simulink model "Event4_2018a"  (R2018a)
settings: Solver=FixedStepDiscrete  StartTime=0.0  StopTime=0.1  FixedStep=0.1  RelTol=1e-3  EnableMultiTasking=on
settings Model: Creator=BEAR  LastModifiedBy=apple
settings SolverCC: AutoInsertRateTranBlk=on
settings DataIOCC: LimitDataPoints=on
settings OptimizationCC: LifeSpan=inf
settings DebuggingCC: AllowSymbolicDim=off  SFUnexpectedBacktrackingDiag=warning  SFNoUnconditionalDefaultTransitionDiag=warning  SFExecutionAtInitializationDiag=none
settings CodeAppCC: StateflowObjectComments=on
settings GRTTargetCC: TargetLangStandard=C89/C90 (ANSI)
settings ConfigComp: CovMetricSettings=dw  CovSaveCumulativeToWorkspaceVar=on  CovSaveSingleToWorkspaceVar=on  CovExternalEMLEnable=off  CovSFcnEnable=off

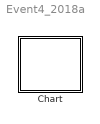
== system Event4_2018a ==
  Chart : Stateflow chart  TreatAsAtomicUnit=on

== stateflow chart Event4_2018a/Chart ==
  state A [parallel]
    settings: executionOrder=1
    state A1
    state A2
      en: fprintf("en_A2")
    (default) -> A1 : {x=-1;}
    A1 -> (junction 40) : E{fprintf("a1");F}
    (junction 40) -> A2 : E{fprintf("a2")}
  state B [parallel]
    settings: executionOrder=2
    state B1
    state B2
      en: fprintf("en_B2")
    (default) -> B1
    B1 -> B2 : {fprintf("b")}/{E;fprintf("tb")}
  state C [parallel]
    settings: executionOrder=3
    state C1
    state C2
      en: fprintf("en_C2")
    (default) -> C1
    C1 -> C2 : F{fprintf("c")}
  data: x local
  events: E local FUNCTION_CALL_EVENT; F local FUNCTION_CALL_EVENT
